simulink model "WEankle_controllerMaarten_TimingPerturb_2018"  (R2018a)
settings: Solver=FixedStepDiscrete  StartTime=0.0  StopTime=inf  FixedStep=sampleTime  RelTol=1e-3
undefined symbols (not defined in the file or in its folder): DiscIntNeverNeededParam, forceplate
libraries: simulink x17, WE2_library x8, dspsigops x6, dspfdesign x3
(part 2 of 3)

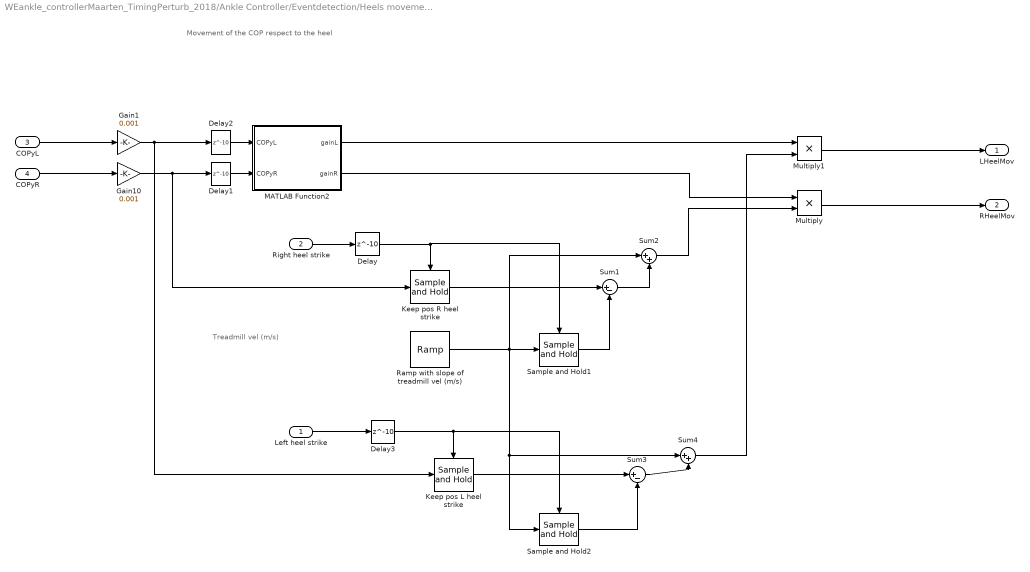
== system WEankle_controllerMaarten_TimingPerturb_2018/Ankle Controller/Eventdetection/Heels movement ==
  note: Movement of the COP respect to the heel
  note: Treadmill vel (m/s)
  Left heel strike : Inport
  Right heel strike : Inport  Port=2
  COPyL : Inport  Port=3
  COPyR : Inport  Port=4
  Delay{,1..3} (4 alike) : Delay  DelayLength=10
  Gain1 : Gain  Gain=0.001
  Gain10 : Gain  Gain=0.001
  Keep pos L heel strike : dspsigops/Sample and Hold  trig=Rising edge  initCond=0  latchinput=off
  Keep pos R heel strike : dspsigops/Sample and Hold  trig=Rising edge  initCond=0  latchinput=off
  MATLAB Function2 : MATLAB Function  TreatAsAtomicUnit=on
  Multiply : Product
  Multiply1 : Product
  Ramp with slope of treadmill vel (m/s) : simulink/Sources/Ramp  slope=-0.56  start=0  InitialOutput=0
  Sample and Hold1 : dspsigops/Sample and Hold  trig=Rising edge  initCond=0  latchinput=off
  Sample and Hold2 : dspsigops/Sample and Hold  trig=Rising edge  initCond=0  latchinput=off
  Sum1 : Sum  Inputs=|+-
  Sum2 : Sum  Inputs=|++
  Sum3 : Sum  Inputs=|+-
  Sum4 : Sum  Inputs=|++
  LHeelMov : Outport  VectorParamsAs1DForOutWhenUnconnected=off
  RHeelMov : Outport  Port=2  VectorParamsAs1DForOutWhenUnconnected=off
  wires:
  Sum2/1 -> Multiply/2
  Delay1/1 -> MATLAB Function2/2(COPyR)
  Ramp with slope of treadmill vel (m/s)/1 -> Sum4/1, Sample and Hold2/1, Sum2/1, Sample and Hold1/1
  Multiply/1 -> RHeelMov/1
  MATLAB Function2/2(gainR) -> Multiply/1
  Keep pos R heel strike/1 -> Sum1/1
  COPyR/1 -> Gain10/1
  Delay/1 -> Keep pos R heel strike/Trigger, Sample and Hold1/Trigger
  Gain10/1 -> Keep pos R heel strike/1, Delay1/1
  Sample and Hold1/1 -> Sum1/2
  Sum1/1 -> Sum2/2
  Right heel strike/1 -> Delay/1
  Delay2/1 -> MATLAB Function2/1(COPyL)
  Gain1/1 -> Delay2/1, Keep pos L heel strike/1
  COPyL/1 -> Gain1/1
  MATLAB Function2/1(gainL) -> Multiply1/1
  Left heel strike/1 -> Delay3/1
  Delay3/1 -> Sample and Hold2/Trigger, Keep pos L heel strike/Trigger
  Keep pos L heel strike/1 -> Sum3/1
  Sample and Hold2/1 -> Sum3/2
  Sum3/1 -> Sum4/2
  Sum4/1 -> Multiply1/2
  Multiply1/1 -> LHeelMov/1

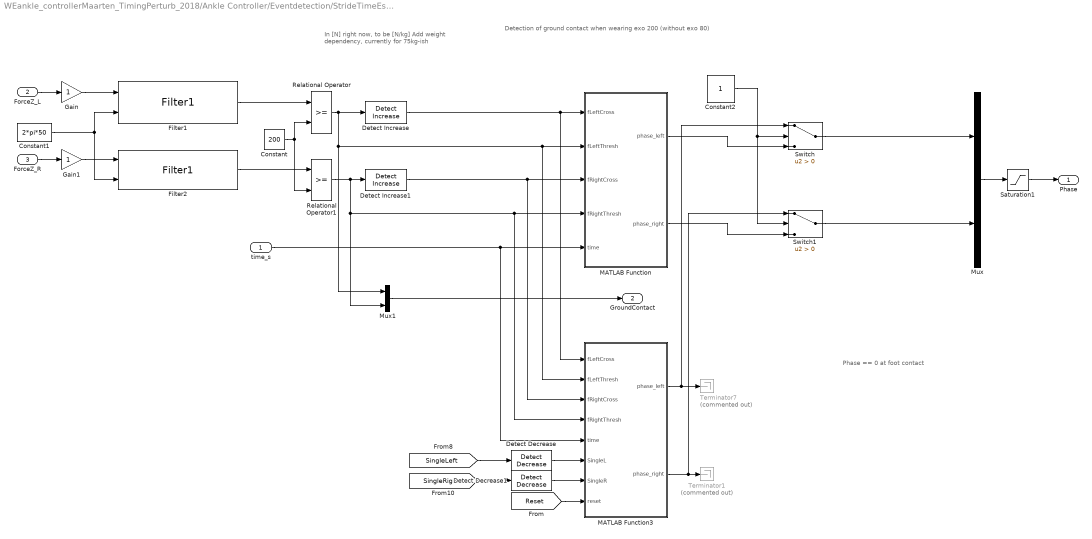
== system WEankle_controllerMaarten_TimingPerturb_2018/Ankle Controller/Eventdetection/StrideTimeEstimator ==
  note: In [N] right now, to be [N/kg]
      | Add weight dependency, currently for 75kg-ish
  note: Detection of ground contact when wearing exo 200 (without exo 80)
  note: Phase == 0 at foot contact
  time_s : Inport
  ForceZ_L : Inport  Port=2
  ForceZ_R : Inport  Port=3
  Constant : Constant  Value=200
  Constant1 : Constant  Value=2*pi*50
  Constant2 : Constant  VectorParams1D=off  SampleTime=-1
  Detect Decrease : simulink/Logic and Bit Operations/Detect Decrease  vinit=0.0  OutDataTypeStr=boolean
  Detect Decrease1 : simulink/Logic and Bit Operations/Detect Decrease  vinit=0.0  OutDataTypeStr=boolean
  Detect Increase : simulink/Logic and Bit Operations/Detect Increase  vinit=0.0  OutDataTypeStr=boolean
  Detect Increase1 : simulink/Logic and Bit Operations/Detect Increase  vinit=0.0  OutDataTypeStr=boolean
  Filter1 : WE2_library/FromActuator/ToJointAngle_rad/FilterFourthOrder/Filter1  sampleTime=sampleTime
  Filter2 : WE2_library/FromActuator/ToJointAngle_rad/FilterFourthOrder/Filter1  sampleTime=sampleTime
  Gain : Gain
  Gain1 : Gain
  MATLAB Function : MATLAB Function  TreatAsAtomicUnit=on
  MATLAB Function3 : MATLAB Function  TreatAsAtomicUnit=on
  Mux : Mux  Inputs=2
  Mux1 : Mux  Inputs=2
  Relational Operator : RelationalOperator  OutDataTypeStr=boolean  RndMeth=Simplest
  Relational Operator1 : RelationalOperator  OutDataTypeStr=boolean  RndMeth=Simplest
  Saturation1 : Saturate  UpperLimit=100  LowerLimit=0
  Switch : Switch  Criteria=u2 > Threshold
  Switch1 : Switch  Criteria=u2 > Threshold
  Terminator1 : Terminator  Commented=on
  Terminator7 : Terminator  Commented=on
  Phase : Outport  VectorParamsAs1DForOutWhenUnconnected=off
  GroundContact : Outport  Port=2  VectorParamsAs1DForOutWhenUnconnected=off
  wires:
  Gain1/1 -> Filter2/1
  Gain/1 -> Filter1/1
  Constant1/1 -> Filter1/2, Filter2/2
  Filter1/1 -> Relational Operator/1
  Filter2/1 -> Relational Operator1/1
  Mux1/1 -> GroundContact/1
  Mux/1 -> Saturation1/1
  Saturation1/1 -> Phase/1
  Switch/1 -> Mux/1
  Detect Increase1/1 -> MATLAB Function3/3(fRightCross), MATLAB Function/3(fRightCross)
  Detect Increase/1 -> MATLAB Function3/1(fLeftCross), MATLAB Function/1(fLeftCross)
  Relational Operator1/1 -> Detect Increase1/1, MATLAB Function3/4(fRightThresh), MATLAB Function/4(fRightThresh), Mux1/2
  Relational Operator/1 -> Detect Increase/1, MATLAB Function3/2(fLeftThresh), MATLAB Function/2(fLeftThresh), Mux1/1
  Constant/1 -> Relational Operator1/2, Relational Operator/2
  time_s/1 -> MATLAB Function3/5(time), MATLAB Function/5(time)
  ForceZ_R/1 -> Gain1/1
  ForceZ_L/1 -> Gain/1
  Detect Decrease/1 -> MATLAB Function3/6(SingleL)
  Detect Decrease1/1 -> MATLAB Function3/7(SingleR)
  [SingleRight] -> Detect Decrease1/1
  [SingleLeft] -> Detect Decrease/1
  MATLAB Function3/1(phase_left) -> Switch/1, Terminator7/1
  MATLAB Function3/2(phase_right) -> Switch1/1, Terminator1/1
  Switch1/1 -> Mux/2
  MATLAB Function/2(phase_right) -> Switch1/3
  MATLAB Function/1(phase_left) -> Switch/3
  Constant2/1 -> Switch1/2, Switch/2
  [Reset] -> MATLAB Function3/8(reset)

== system WEankle_controllerMaarten_TimingPerturb_2018/Ankle Controller/Eventdetection/Subsystem ==
  In1 : Inport
  Constant : Constant  Value=5
  Delay2 : Delay  DelayLength=1
  Lowpass Filter2 : dspfdesign/Lowpass Filter  FilterType=IIR  DesignForMinimumOrder=on  FilterOrder=50  PassbandFrequency=40  StopbandFrequency=50  PassbandRipple=0.1  StopbandAttenuation=40  InheritSampleRate=off  SampleRate=1000  SimulateUsing=Interpreted execution  roundingMode=Floor  coeffsDataTypeStr=fixdt(1,16)
  MATLAB Function : MATLAB Function  TreatAsAtomicUnit=on
  Rate Transition : RateTransition
  Out1 : Outport  VectorParamsAs1DForOutWhenUnconnected=off
  wires:
  MATLAB Function/1(y) -> Out1/1
  Rate Transition/1 -> Lowpass Filter2/1
  Constant/1 -> MATLAB Function/4(th)
  Lowpass Filter2/1 -> MATLAB Function/1(f)  "prev"
  Delay2/1 -> MATLAB Function/3(nf_1)
  In1/1 -> Delay2/1, MATLAB Function/2(nf), Rate Transition/1

== system WEankle_controllerMaarten_TimingPerturb_2018/Ankle Controller/Eventdetection/Subsystem1 ==
  In1 : Inport
  Constant : Constant  Value=5
  Delay2 : Delay  DelayLength=1
  Lowpass Filter2 : dspfdesign/Lowpass Filter  FilterType=IIR  DesignForMinimumOrder=on  FilterOrder=50  PassbandFrequency=40  StopbandFrequency=50  PassbandRipple=0.1  StopbandAttenuation=40  InheritSampleRate=off  SampleRate=1000  SimulateUsing=Interpreted execution  roundingMode=Floor  coeffsDataTypeStr=fixdt(1,16)
  MATLAB Function : MATLAB Function  TreatAsAtomicUnit=on
  Rate Transition : RateTransition
  Out1 : Outport  VectorParamsAs1DForOutWhenUnconnected=off
  wires:
  MATLAB Function/1(y) -> Out1/1
  Rate Transition/1 -> Lowpass Filter2/1
  Constant/1 -> MATLAB Function/4(th)
  Lowpass Filter2/1 -> MATLAB Function/1(f)  "prev"
  Delay2/1 -> MATLAB Function/3(nf_1)
  In1/1 -> Delay2/1, MATLAB Function/2(nf), Rate Transition/1

== system WEankle_controllerMaarten_TimingPerturb_2018/Ankle Controller/COMverror and perturbation/COMvError/Data lost detection ==
  note: Assuming no data lost
  Input signal : Inport
  ErrorIn : Inport  Port=2
  Delay : Delay  DelayLength=1
  Delay1 : Delay  DelayLength=1
  Gain1 : Gain  Gain=0
  Gain2 : Gain  Gain=100
  MATLAB Function1 : MATLAB Function  TreatAsAtomicUnit=on
  MATLAB Function2 : MATLAB Function  TreatAsAtomicUnit=on
  New error : Outport  VectorParamsAs1DForOutWhenUnconnected=off
  DataLost : Outport  Port=2  VectorParamsAs1DForOutWhenUnconnected=off
  avoid : Outport  Port=3  VectorParamsAs1DForOutWhenUnconnected=off
  wires:
  MATLAB Function2/2(avoid) -> avoid/1
  ErrorIn/1 -> MATLAB Function2/3(ErrorIn)
  Delay/1 -> MATLAB Function1/2(u_1)
  MATLAB Function2/1(ErrorOut) -> New error/1  "New error"
  Delay1/1 -> MATLAB Function2/2(DataLost_1)
  Input signal/1 -> MATLAB Function1/1(u), Delay/1
  MATLAB Function1/1(y) -> Gain1/1
  Gain2/1 -> DataLost/1  "DataLost"
  Gain1/1 -> Delay1/1, MATLAB Function2/1(DataLost), Gain2/1  "DataLost"

== system WEankle_controllerMaarten_TimingPerturb_2018/Ankle Controller/COMverror and perturbation/COMvError/PertDetection ==
  PertFromError : Inport
  PertFromInputSignal : Inport  Port=2
  avoid : Inport  Port=3
  Delay : Delay  DelayLength=1
  Detect Increase : simulink/Logic and Bit Operations/Detect Increase  vinit=0  OutDataTypeStr=boolean
  MATLAB Function1 : MATLAB Function  TreatAsAtomicUnit=on
  MATLAB Function2 : MATLAB Function  TreatAsAtomicUnit=on
  PertDetect : Outport  VectorParamsAs1DForOutWhenUnconnected=off
  wires:
  Detect Increase/1 -> MATLAB Function1/4(StartPertFromError)
  Delay/1 -> MATLAB Function2/2(Pert_1)
  MATLAB Function1/1(PertDetect) -> Delay/1, MATLAB Function2/1(Pert)
  PertFromInputSignal/1 -> MATLAB Function1/2(PertFromInput)
  MATLAB Function2/1(PertDetect) -> PertDetect/1
  PertFromError/1 -> MATLAB Function1/1(PertFromError), Detect Increase/1
  avoid/1 -> MATLAB Function1/3(avoid)

== system WEankle_controllerMaarten_TimingPerturb_2018/Ankle Controller/COMverror and perturbation/COMvError/Signal learner ==
  note: To convert pos to vel
  note: Excluding for the average those steps where a perturbation happened.
      | The threshold to calculate which steps where perturbed is taken as the
      | mean of maximums in previous steps. Avoiding DataLost and false Triggers
  Signaltime : Inport
  trigger : Inport  Port=2
  xPosCOM : Inport  Port=3
  Constant : Constant  Value=6
  Constant1 : Constant  Value=1.5
  Discrete Derivative1 : simulink/Discrete/Discrete Derivative  gainval=1.0  ICPrevScaledInput=0.0  OutMin=[]  OutMax=[]  OutDataType=fixdt(1, 16)  OutScaling=2^-10  DoSatur=off
  Lowpass Filter2 : dspfdesign/Lowpass Filter  FilterType=IIR  DesignForMinimumOrder=on  FilterOrder=50  PassbandFrequency=5  StopbandFrequency=50  PassbandRipple=0.1  StopbandAttenuation=40  InheritSampleRate=off  SampleRate=1000  SimulateUsing=Interpreted execution  roundingMode=Floor  coeffsDataTypeStr=fixdt(1,16)
  MATLAB Function : MATLAB Function  TreatAsAtomicUnit=on
  Rate Transition : RateTransition
  Sum : Sum  Inputs=|+-
  original : Outport  VectorParamsAs1DForOutWhenUnconnected=off
  error : Outport  Port=2  VectorParamsAs1DForOutWhenUnconnected=off
  Input filtered : Outport  Port=3  VectorParamsAs1DForOutWhenUnconnected=off
  learned : Outport  Port=4  VectorParamsAs1DForOutWhenUnconnected=off
  Perturbation detected FromInput : Outport  Port=5  VectorParamsAs1DForOutWhenUnconnected=off
  ShutDown : Outport  Port=6  VectorParamsAs1DForOutWhenUnconnected=off
  tag scope: m=global, n=global, n_strides=global, stride_duration=global
  wires:
  MATLAB Function/7(ShutDown) -> ShutDown/1
  [DataLost] -> MATLAB Function/7(DataLost)  "DataLost"
  Constant1/1 -> MATLAB Function/6(threshPert)
  MATLAB Function/6(perturbation) -> Perturbation detected FromInput/1
  trigger/1 -> MATLAB Function/3(trigger)
  Sum/1 -> error/1  "error"
  Signaltime/1 -> MATLAB Function/2(t)
  MATLAB Function/5(output_duration_) -> [stride_duration]  "stride_duration"
  Constant/1 -> MATLAB Function/5(n_rep)
  MATLAB Function/4(m_) -> [m]  "m"
  MATLAB Function/1(signal_learned) -> Sum/2, learned/1  "learned"
  MATLAB Function/2(n_strides_) -> [n_strides]  "n_strides"
  MATLAB Function/3(n_) -> [n]  "n"
  Lowpass Filter2/1 -> Sum/1, Input filtered/1, MATLAB Function/4(signal)  "prev"
  xPosCOM/1 -> Discrete Derivative1/1  "original"
  Discrete Derivative1/1 -> Rate Transition/1  "original"
  Rate Transition/1 -> original/1, Lowpass Filter2/1
  [Reset] -> MATLAB Function/1(reset)

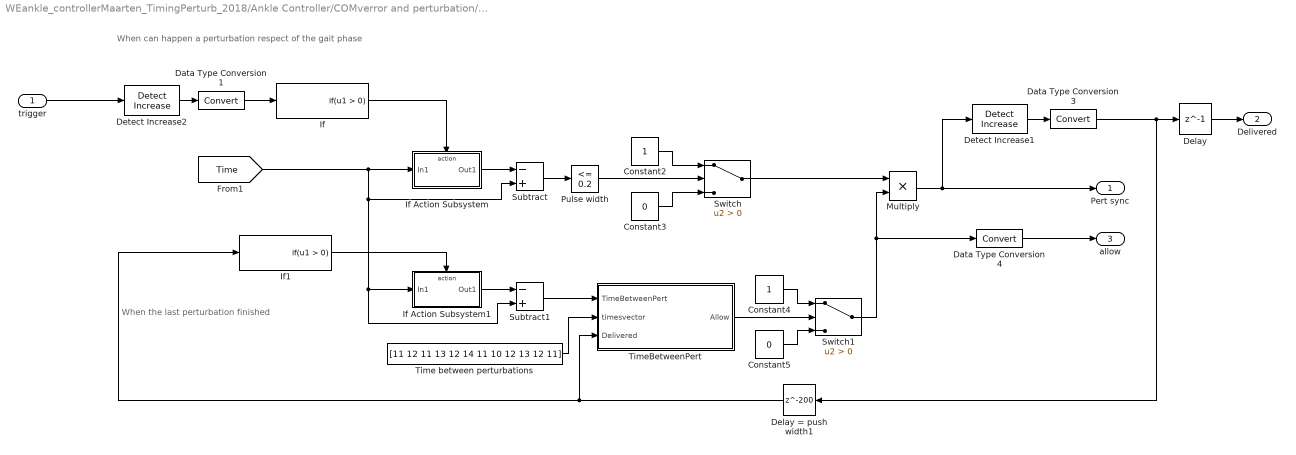
== system WEankle_controllerMaarten_TimingPerturb_2018/Ankle Controller/COMverror and perturbation/TriggerPerturbation/Perturbation sync gait phase1 ==
  note: When the last perturbation finished
  note: When can happen a perturbation respect of the gait phase
  trigger : Inport
  Constant2 : Constant
  Constant3 : Constant  Value=0
  Constant4 : Constant
  Constant5 : Constant  Value=0
  Data Type Conversion1 : DataTypeConversion
  Data Type Conversion3 : DataTypeConversion
  Data Type Conversion4 : DataTypeConversion
  Delay : Delay  DelayLength=1
  Delay = push width1 : Delay  DelayLength=200  InitialCondition=0
  Detect Increase1 : simulink/Logic and Bit Operations/Detect Increase  vinit=0  OutDataTypeStr=boolean
  Detect Increase2 : simulink/Logic and Bit Operations/Detect Increase  vinit=0  OutDataTypeStr=boolean
  If : If  ShowElse=off
  If Action Subsystem : Subsystem  TreatAsAtomicUnit=on
  If Action Subsystem1 : Subsystem  TreatAsAtomicUnit=on
  If1 : If  ShowElse=off
  Multiply : Product
  Pulse width : simulink/Logic and Bit Operations/Compare To Constant  relop=<=  const=0.2  OutDataTypeStr=boolean
  Subtract : Sum  Inputs=-+
  Subtract1 : Sum  Inputs=-+
  Switch : Switch  Criteria=u2 > Threshold
  Switch1 : Switch  Criteria=u2 > Threshold
  Time between perturbations : Constant  Value=[11 12 11 13 12 14 11 10 12 13 12 11]
  TimeBetweenPert : MATLAB Function  TreatAsAtomicUnit=on
  Pert sync : Outport  VectorParamsAs1DForOutWhenUnconnected=off
  Delivered : Outport  Port=2  VectorParamsAs1DForOutWhenUnconnected=off
  allow : Outport  Port=3  VectorParamsAs1DForOutWhenUnconnected=off
  wires:
  Time between perturbations/1 -> TimeBetweenPert/2(timesvector)
  Subtract1/1 -> TimeBetweenPert/1(TimeBetweenPert)
  TimeBetweenPert/1(Allow) -> Switch1/2
  Data Type Conversion4/1 -> allow/1
  Delay/1 -> Delivered/1
  Data Type Conversion3/1 -> Delay/1, Delay = push width1/1
  Delay = push width1/1 -> If1/1, TimeBetweenPert/3(Delivered)
  If1/1 -> If Action Subsystem1/Action
  Constant3/1 -> Switch/3
  If/1 -> If Action Subsystem/Action
  Constant2/1 -> Switch/1
  [Time] -> Subtract1/2, If Action Subsystem1/1(In1), Subtract/2, If Action Subsystem/1(In1)
  Constant5/1 -> Switch1/3
  Pulse width/1 -> Switch/2
  Multiply/1 -> Detect Increase1/1, Pert sync/1
  If Action Subsystem/1(Out1) -> Subtract/1
  If Action Subsystem1/1(Out1) -> Subtract1/1
  trigger/1 -> Detect Increase2/1
  Subtract/1 -> Pulse width/1
  Switch/1 -> Multiply/1
  Switch1/1 -> Multiply/2, Data Type Conversion4/1
  Detect Increase2/1 -> Data Type Conversion1/1
  Data Type Conversion1/1 -> If/1
  Constant4/1 -> Switch1/1
  Detect Increase1/1 -> Data Type Conversion3/1

== system WEankle_controllerMaarten_TimingPerturb_2018/Ankle Controller/Eventdetection/COP detection (treadmill)/Get_COPL ==
  note: COPx
  note: COPy
  grf : Inport
  Enable : EnablePort  StatesWhenEnabling=reset
  Demux1 : Demux  Outputs=3
  Divide : Product  Inputs=*/
  Divide1 : Product  Inputs=*/
  Gain : Gain  Gain=-1
  LEFT Mx My Fz : Selector  InputPortWidth=6  IndexOptions=Index vector (dialog)  Indices=[4 5 3]  OutputSizes=1
  Mux : Mux  Inputs=2
  COPL : Outport  OutputWhenDisabled=reset  InitialOutput=0  VectorParamsAs1DForOutWhenUnconnected=off
  wires:
  grf/1 -> LEFT Mx My Fz/1
  LEFT Mx My Fz/1 -> Demux1/1
  Demux1/2 -> Gain/1  "My"
  Gain/1 -> Divide/1
  Demux1/3 -> Divide1/2, Divide/2  "Fz"
  Demux1/1 -> Divide1/1  "Mx"
  Divide/1 -> Mux/1
  Divide1/1 -> Mux/2
  Mux/1 -> COPL/1

== system WEankle_controllerMaarten_TimingPerturb_2018/Ankle Controller/Eventdetection/COP detection (treadmill)/Get_COPR ==
  note: COPx
  note: COPy
  grf : Inport
  Enable : EnablePort  StatesWhenEnabling=reset
  Demux1 : Demux  Outputs=3
  Divide : Product  Inputs=*/
  Divide1 : Product  Inputs=*/
  Gain : Gain  Gain=-1
  Mux : Mux  Inputs=2
  RIGHT Mx My Fz : Selector  InputPortWidth=6  IndexOptions=Index vector (dialog)  Indices=[4 5 3]  OutputSizes=1
  COPR : Outport  OutputWhenDisabled=reset  InitialOutput=0  VectorParamsAs1DForOutWhenUnconnected=off
  wires:
  grf/1 -> RIGHT Mx My Fz/1
  RIGHT Mx My Fz/1 -> Demux1/1
  Demux1/2 -> Gain/1  "My"
  Gain/1 -> Divide/1
  Demux1/3 -> Divide1/2, Divide/2  "Fz"
  Demux1/1 -> Divide1/1  "Mx"
  Divide/1 -> Mux/1
  Divide1/1 -> Mux/2
  Mux/1 -> COPR/1

== system WEankle_controllerMaarten_TimingPerturb_2018/Ankle Controller/COMverror and perturbation/TriggerPerturbation/Perturbation sync gait phase1/If Action Subsystem ==
  In1 : Inport
  Action Port : ActionPort
  Out1 : Outport  VectorParamsAs1DForOutWhenUnconnected=off
  wires:
  In1/1 -> Out1/1

== system WEankle_controllerMaarten_TimingPerturb_2018/Ankle Controller/COMverror and perturbation/TriggerPerturbation/Perturbation sync gait phase1/If Action Subsystem1 ==
  In1 : Inport
  Action Port : ActionPort
  Out1 : Outport  VectorParamsAs1DForOutWhenUnconnected=off
  wires:
  In1/1 -> Out1/1

== matlab function WEankle_controllerMaarten_TimingPerturb_2018/Ankle Controller/Eventdetection/StrideTimeEstimator/MATLAB Function ==
  data: fLeftCross input; fLeftThresh input; phase_left output; fRightCross input; fRightThresh input; time input; phase_right output
function [phase_left, phase_right] = fcn(fLeftCross, fLeftThresh, fRightCross, fRightThresh, time)

persistent time_heel2heel_right
persistent time_heellast_right
persistent tdm_right
persistent time_heel2heel_left
persistent time_heellast_left
persistent tdm_left

if(isempty(time_heel2heel_left))
   time_heel2heel_right = zeros(4,1);
   time_heellast_right = -1e5;
   tdm_right = 0.1;
   
   time_heel2heel_left = zeros(4,1);
   time_heellast_left = -1e5;
   tdm_left = 0.1;
end
%% left
phase_left = (time - time_heellast_left)/(tdm_left+eps)*100;
if(fLeftCross~=0||(phase_left>100&&fLeftThresh==1))
    td_new  = time - time_heellast_left;
    if((td_new>0.8*tdm_left)||any(time_heel2heel_left>10))
        time_heellast_left = time;
        time_heel2heel_left(2:end) = time_heel2heel_left(1:end-1);
        time_heel2heel_left(1) = td_new;
        tdm_left = mean(time_heel2heel_left);
    end
end


%% right
phase_right = (time - time_heellast_right)/(tdm_right+eps)*100;
if(fRightCross~=0||(phase_right>100&&fRightThresh==1))
    td_new  = time - time_heellast_right;
    if((td_new>0.8*tdm_right)||any(time_heel2heel_right>10))
        time_heellast_right = time;
        time_heel2heel_right(2:end) = time_heel2heel_right(1:end-1);
        time_heel2heel_right(1) = td_new;
        tdm_right = mean(time_heel2heel_right);
    end
end

== matlab function WEankle_controllerMaarten_TimingPerturb_2018/Ankle Controller/Eventdetection/COP detection (treadmill)/MATLAB Function1 ==
  data: x input; y output; OmegaFilter input; sampleTime input
function y = Filter2ndOrder(x, OmegaFilter, sampleTime)
%#codegen

persistent yd_prev y_prev;
if isempty(yd_prev)
    yd_prev = zeros(6,1); 
    y_prev = zeros(6,1);  %Derivative of the above signal
end

% Do 2nd order filtering with given omega and zeta=0.7; input of filter
% is vel_inc_sampleTime_unfilt; output is y (we assign to vel_inc_s
% later). 
if OmegaFilter==0 || isinf(OmegaFilter)
    y = x;
    y_prev = y;
    yd_prev = zeros(6,1); 
else
    zeta = 0.7;
    ydd = OmegaFilter^2 * (x - y_prev) - 2*zeta*OmegaFilter* yd_prev;
    yd = yd_prev + ydd * sampleTime;
    y = y_prev + yd * sampleTime;

    y_prev = y; yd_prev = yd;
end

== matlab function WEankle_controllerMaarten_TimingPerturb_2018/Ankle Controller/MATLAB Function5 ==
  data: e0 input; G input; SolGains output; COMd input
function SolGains  = CombineSoleusGains(e0,G,COMd)
% input arguments:

SolGains = [e0; G; COMd];

== matlab function WEankle_controllerMaarten_TimingPerturb_2018/ForcePlate/Calibration/MATLAB Function ==
  data: left input; left_calib output; right input; start input; right_calib output; caltime_s input
function [left_calib, right_calib] = calibrateOffset(left, right, start, caltime_s)
persistent calibrated
persistent offcum_left
persistent offcum_right
persistent counter
persistent nosamp

if(isempty(calibrated))
   calibrated = false;
   offcum_left = left*0;
   offcum_right = right*0;
   counter = 0;
   nosamp = max(1, floor(caltime_s*1000));
end

if(start == 1)
    counter = 0;
    calibrated = false;
    offcum_left = left*0;
    offcum_right = right*0;
    nosamp = max(1, floor(caltime_s*1000));
end

if(calibrated)
    left_calib = left - offcum_left;
    right_calib = right - offcum_right;
else
    if(~calibrated)
        counter = counter + 1;
        offcum_left = offcum_left + left/(nosamp);
        offcum_right = offcum_right + right/(nosamp);
        if(counter >= nosamp)
            calibrated = true;
        end
    end
    left_calib = left;
    right_calib = right;
end

== matlab function WEankle_controllerMaarten_TimingPerturb_2018/Ankle Controller/Eventdetection/COP detection (treadmill)/MATLAB Function2 ==
  data: x input; y output; OmegaFilter input; sampleTime input
function y = Filter2ndOrder(x, OmegaFilter, sampleTime)
%#codegen

persistent yd_prev y_prev;
if isempty(yd_prev)
    yd_prev = zeros(6,1); 
    y_prev = zeros(6,1);  %Derivative of the above signal
end

% Do 2nd order filtering with given omega and zeta=0.7; input of filter
% is vel_inc_sampleTime_unfilt; output is y (we assign to vel_inc_s
% later). 
if OmegaFilter==0 || isinf(OmegaFilter)
    y = x;
    y_prev = y;
    yd_prev = zeros(6,1); 
else
    zeta = 0.7;
    ydd = OmegaFilter^2 * (x - y_prev) - 2*zeta*OmegaFilter* yd_prev;
    yd = yd_prev + ydd * sampleTime;
    y = y_prev + yd * sampleTime;

    y_prev = y; yd_prev = yd;
end

== matlab function WEankle_controllerMaarten_TimingPerturb_2018/Ankle Controller/COMverror and perturbation/TriggerPerturbation/Perturbation sync gait phase1/TimeBetweenPert ==
  data: TimeBetweenPert input; timesvector input; Allow output; Delivered input
function Allow = fcn(TimeBetweenPert,timesvector,Delivered)
% To randomize the time between perturbations (min 6s)
persistent i 
persistent TimeSelector 
persistent flagfirst %flag to indicate first time
if isempty(i)
    i = 1;
    flagfirst = 1;
end
if Delivered == 1 && ~flagfirst %Perturbation delivered. Go to next element of timesVector avoiding a false entrance the first time
    i = i+1;
end
%% Assign new time
len = length(timesvector);
if i > len %reset the index when all perturbations from the vector are done
    i = 1;
end
TimeSelector = timesvector(i);

if TimeSelector < 6
    TimeSelector = 6;
end
%% Allow new perturbation or not
if TimeBetweenPert >= TimeSelector
    Allow = 1;
else
    Allow = 0;
end
%%
flagfirst = 0;

== matlab function WEankle_controllerMaarten_TimingPerturb_2018/Ankle Controller/Eventdetection/Subsystem/MATLAB Function ==
  data: f input; y output; nf input; nf_1 input; th input
function y = fcn(f,nf,nf_1,th)

maxCounter = 200; %time to wait in zero
persistent counter
persistent out
if isempty(counter)
    counter = maxCounter+1;
    out = f;
end

if (nf == 0) && (nf_1 < -50)
    out = 0;
    counter = 0;
else
    counter = counter+1;
    if counter > maxCounter
        if (f > -th) && (f < th) && (nf == 0)
            out = 0;
        else
            out = f;
        end
    end
end

y = out;

== matlab function WEankle_controllerMaarten_TimingPerturb_2018/Ankle Controller/Eventdetection/StrideTimeEstimator/MATLAB Function3 ==
  data: fLeftCross input; fLeftThresh input; phase_left output; fRightCross input; fRightThresh input; time input; phase_right output; SingleL input; SingleR input; reset input
function [phase_left, phase_right] = fcn(fLeftCross, fLeftThresh, fRightCross, fRightThresh, time, SingleL, SingleR, reset)

persistent time_heel2heel_right
persistent time_heellast_right
persistent tdm_right
persistent time_heel2heel_left
persistent time_heellast_left
persistent tdm_left
persistent  phase_left2
persistent  phase_right2

if(isempty(time_heel2heel_left) || reset==1)
   time_heel2heel_right = zeros(4,1);
   time_heellast_right = -1e5;
   tdm_right = 0.1;
   
   time_heel2heel_left = zeros(4,1);
   time_heellast_left = -1e5;
   tdm_left = 0.1;
   
    phase_left2 = 0; %Used to reset the left phase when prepositioning of left leg is detected (SingleL 1 to 0)
    phase_right2 = 0; %Used to reset the right phase when prepositioning of right leg is detected (SingleR 1 to 0)
end
%% left
phase_left = (time - time_heellast_left)/(tdm_left+eps)*100 - phase_left2;
% if(fLeftCross~=0||(phase_left>100&&fLeftThresh==1))

if(SingleR)
    phase_left2 = phase_left;
end
if((fLeftCross~=0||(phase_left>100&&fLeftThresh==1)))
    td_new  = time - time_heellast_left;
    phase_left2 = 0;
    if((td_new>0.8*tdm_left)||any(time_heel2heel_left>10))
        time_heellast_left = time;
        time_heel2heel_left(2:end) = time_heel2heel_left(1:end-1);
        time_heel2heel_left(1) = td_new;
        tdm_left = mean(time_heel2heel_left);
    end
end


%% right
phase_right = (time - time_heellast_right)/(tdm_right+eps)*100 - phase_right2;
% if(fRightCross~=0||(phase_right>100&&fRightThresh==1))
if(SingleL)
    phase_right2 = phase_right;
end
if(fRightCross~=0||(phase_right>100&&fRightThresh==1))
    td_new  = time - time_heellast_right;
    phase_right2 = 0;
    if((td_new>0.8*tdm_right)||any(time_heel2heel_right>10))
        time_heellast_right = time;
        time_heel2heel_right(2:end) = time_heel2heel_right(1:end-1);
        time_heel2heel_right(1) = td_new;
        tdm_right = mean(time_heel2heel_right);
    end
end

== matlab function WEankle_controllerMaarten_TimingPerturb_2018/Merge 32 bit to double/MATLAB Function ==
  data: time_0 input; unix_time output double size=1; time_1 input int32 size=1
function unix_time  = fcn(time_0, time_1)

% Convert both integers to double, scale up the most significant part and
% add them together.
% The epoch is also moved from 1601 to 1970, this is done in the integer
% part.

double_0 = double(time_0);
double_1 = double(time_1 - int32(27111902));
unix_time = (double_1 * 2^32 + double_0 - 3577643008.0) * 1.0e-7;

% A 64 bit integer does not exist in Simulink 2018b. Casting is also not
% possible, otherwise the following would work:
% time_64bit = typecast([time_0, time_1], 'int64');
% unix_time = double(time_64bit);

end

== matlab function WEankle_controllerMaarten_TimingPerturb_2018/Ankle Controller/COMverror and perturbation/TriggerPerturbation/MakeVect ==
  data: u input; y output
function y = fcn(u)

y = [u, u, u, u, u];

== matlab function WEankle_controllerMaarten_TimingPerturb_2018/Ankle Controller/COMDLimits ==
  data: comd input; comd_out output
function comd_out = COMd_bounds(comd)


tresh = 200; % 200mm/s

if abs(comd)<tresh    
    comd = 0;
end


comd_out = comd;

== matlab function WEankle_controllerMaarten_TimingPerturb_2018/Ankle Controller/Eventdetection/Heels movement/MATLAB Function2 ==
  data: gainL output; COPyL input; gainR output; COPyR input
function [gainL,gainR] = Stance(COPyL,COPyR)
%#codegen
if COPyR == 0
    gainR = 0;
else
    gainR = 1;
end

if COPyL == 0
    gainL = 0;
else
    gainL = 1;
end

end

== matlab function WEankle_controllerMaarten_TimingPerturb_2018/Ankle Controller/COMverror and perturbation/TriggerPerturbation/PushOrPull ==
  data: Perturb input; vectorPushPull input; NewPert output; Delivered input
function NewPert = fcn(Perturb,vectorPushPull,Delivered)
% To randomize pushes and pulls
persistent i 
persistent Selector 
persistent flagfirst %flag to indicate first time
if isempty(i)
    i = 1;
    flagfirst = 1;
end
if Delivered == 1 && ~flagfirst %Perturbation delivered. Go to next element of timesVector avoiding a false entrance the first time
    i = i+1;
end
%%
len = length(vectorPushPull);
if i > len %reset the index when all perturbations from the vector are done
    i = 1;
end
Selector = vectorPushPull(i);

if Selector < -1
    Selector = -1;
elseif Selector > 1
    Selector = 1;
end
%% 
NewPert = Selector*Perturb;
%%
flagfirst = 0;

== matlab function WEankle_controllerMaarten_TimingPerturb_2018/Ankle Controller/COMverror and perturbation/COMvError/MATLAB Function1 ==
  data: ShutDown input; PertDetect input; TriggerPush output
function TriggerPush = fcn(ShutDown,PertDetect)
if ShutDown == 0
    TriggerPush = PertDetect;
else
    TriggerPush = 0;
end

== matlab function WEankle_controllerMaarten_TimingPerturb_2018/Ankle Controller/COMverror and perturbation/COMvError/Signal learner/MATLAB Function ==
  data: reset input; t input; trigger input; signal input; signal_learned output; n_strides_ output; n_ output; m_ output; output_duration_ output; n_rep input; perturbation output; threshPert input; DataLost input; ShutDown output
function [signal_learned,n_strides_,n_,m_,output_duration_,perturbation,ShutDown] = signal_learner(reset,t,trigger,signal,n_rep,threshPert,DataLost)
%     n_rep = how many signals period will be averaged
n_storage = 2000; %stored signal will be 2000 elements long. playback will be interpolated
n_buffer_size = 4000; %can maximally read 4000;
perturbation = 0;
ShutDown = 0; %No trigger the controller if DataLost or if we are in the first n_rep strides
persistent n %elements of vector
persistent n_strides % total number of strides
persistent m %Pointer for recording each stride in buffer (1:n_rep)
persistent t0 % moment in time of last stride
persistent last_buffer
persistent output_signal_buffer
persistent output_signal
persistent output_duration
persistent output_duration_buffer
persistent maximums
persistent MaxAver
persistent LastTrigger



if isempty(n)
    n = 1;
    m = 1;
    t0 = 0;
    last_buffer = zeros(1,n_buffer_size);
    output_signal_buffer = zeros(n_rep,n_storage);
    output_signal = zeros(1,n_storage);
    output_duration_buffer = zeros(n_rep,1);
    n_strides = 0;
    output_duration = 1;
    % Added Cristina
    maximums = 200*ones(n_rep,1); %to store the maximums of previous steps
    MaxAver = 200; % This number multiplied by 1.5 is the one above which a perturbation is supposed to happen,
    %     and thereby, that step will be excluded to calculate the mean
    LastTrigger = 0;
end

dtStride = t-LastTrigger;
if trigger
    LastTrigger = t;
end

if dtStride <0.1 || dtStride > 4
    reset = 1;
end



if ~DataLost && ~reset
    t_rel = t-t0;
    if (trigger && t_rel > 0.1) %if trigger happens, note down the absolute time when that was
        n_strides = n_strides+1; %counting number of strides
        last_stride_duration = t-t0;
        
        t0 = t; %Reset the moment when the last stride happened
        %% Added Cristina
        % See if there was a perturbation in the last step
        Perturbation = 0; % Init perturbation in the last step
%         leng = length(last_buffer(1:min([n,n_buffer_size])));
%         for i = 1:leng
%             element = last_buffer(i);
%             if element > 1.5*MaxAver % A perturbation was detected in the last step
%                 Perturbation = 1;
%             end
%         end
        
        %% Changed Cristina
        enter = 1;
%         if n_strides >= 3
%             if (last_stride_duration > 0.5*output_duration)% to avoid false triggers
%                 enter = 1;
%             else
%                 enter = 0;
%             end
%         else
%             enter = 1;
%         end
        if (last_stride_duration > 0) && enter % otherwise failure at start or false trigger  
            % If there was no perturbation, take that step into account.
            % Otherwise, exclude it
            if ~Perturbation %in the last step
                %interpolate regardless of last duration to n_storage elements
%                 if n == 1
%                     n = n+1;
%                 end
                output_signal_buffer(m,:) = ...
                    interp1(...
                    linspace(0,last_stride_duration,n),... %vector of n elements
                    last_buffer(1:min([n,n_buffer_size])),... %only read up to incl. n elements, if bigger than n_buffer size, then we need to limit.
                    linspace(0,last_stride_duration,n_storage)); %remap that to a new 'x' with n_storage elements
                output_signal = mean(output_signal_buffer); %averages over n_rep stored signals
                
                output_duration_buffer(m) = last_stride_duration;
                output_duration = mean(output_duration_buffer); %duration is average of last n_rep times
                
                maximums(m) = max(last_buffer(1:min([n,n_buffer_size]))); %store the new maximum of current step
                MaxAver = mean(maximums); %calculate the average of maximums found in the last n_rep
                
                m = m+1;
                if m > n_rep
                    m = 1;
                end
            end
            if (n_strides <= n_rep)
                output_duration = last_stride_duration;
            end
            %last_buffer = zeros() %is not required due to 1:n
            n = 1;
        end
    end
end
if ~DataLost && ~reset
    %% process input
    t_rel = t-t0;
    last_buffer(min([n n_buffer_size])) = signal;
    
    %% generate output
    fractional_index = t_rel/output_duration * (n_storage-1);
    rounded_index = min([1+floor(fractional_index),n_storage]); %cannot overflow
    fraction = 1+fractional_index - rounded_index;
    
    %linearly interpolate
    if (rounded_index >= n_storage - 1)
        signal_learned = output_signal(n_storage-1);
    else
        signal_learned = output_signal(rounded_index)*(1-fraction) + output_signal(rounded_index+1)*fraction;
    end
    
    %debug output
    n_strides_ = n_strides;
    n_ = n;
    m_ = m;
    output_duration_ = output_duration;
    if signal > threshPert*MaxAver
        perturbation = 1;
    end
else
    %debug output
    n_strides_ = n_strides;
    n_ = n;
    m_ = m;
    output_duration_ = output_duration;
    perturbation = 0;
    signal_learned = 0;
end

%do not output anything learned in first n_rep strides.
if (n_strides <= n_rep) || DataLost || reset
    signal_learned = 0;
    output_duration_ = 0;%last_stride_duration;
    ShutDown = 1;
end
if ~DataLost && ~reset
    %shift signal storage pointer, avoid overflow
    n = n+1;
else
    n = 1;
end
end

== matlab function WEankle_controllerMaarten_TimingPerturb_2018/Ankle Controller/COMverror and perturbation/COMvError/Data lost detection/MATLAB Function1 ==
  data: u input; y output; u_1 input
function y = fcn(u,u_1)
% input signal u = xVelCOM
% output y = data lost detection (1 or 0)
y = 0;
if u == u_1 % The new data is equal to the previous one --> See how Qualisys will send it since NaN is not supported
    y = 1; % Data lost
else
    y = 0; % Data good
end

== matlab function WEankle_controllerMaarten_TimingPerturb_2018/Ankle Controller/COMverror and perturbation/COMvError/Data lost detection/MATLAB Function2 ==
  data: DataLost input; DataLost_1 input; ErrorOut output; ErrorIn input; avoid output
function [ErrorOut,avoid] = fcn(DataLost,DataLost_1,ErrorIn)
% ErrorOut is the new error corrected when data lost

maxCounter = 1500; %time to wait after a DataLost detection to let the controller works again (1.5s)
persistent counter
if isempty(counter)
    counter = maxCounter+1;
end

ErrorOut = ErrorIn;
avoid = 0;

if DataLost == 1 % Data lost
    ErrorOut = 0; 
    avoid = 1;
elseif DataLost == 0 && DataLost_1 == 1 % Data just recovered after a loss
    counter = 1;
    ErrorOut = 0; 
    avoid = 1;
elseif DataLost == 0 && DataLost_1 ~= 1 % Good data
    if counter <= maxCounter % Wait 1.5s after data has been recovered to generate the newError
        ErrorOut = 0;
        avoid = 1;
        counter = counter + 1;
    else
        ErrorOut = ErrorIn;
        avoid = 0;
    end
end

== matlab function WEankle_controllerMaarten_TimingPerturb_2018/Ankle Controller/COMverror and perturbation/COMvError/PerturbationDetectionFromError ==
  data: t input; trigger input; signal input; n_rep input; push output; maxAver output; rangeAver output; threshPert input; DataLost input
function [push,maxAver,rangeAver] = PerturbationDetectionFromError(t,trigger,signal,n_rep,threshPert,DataLost)
    n_buffer_size = 4000; %can maximally read 4000;
    push = 0; 
    
    persistent n %elements of vector
    persistent n_strides % total number of strides
    persistent m %Pointer for recording each stride in buffer (1:n_rep)
    persistent t0 % moment in time of last stride
    persistent last_buffer
    persistent maximums
    persistent MaxAver
    persistent minimums
    persistent MinAver
    persistent RangeAver

    if isempty(n)
       n = 1;
       m = 1;
       t0 = 0;
       last_buffer = zeros(1,n_buffer_size);
       n_strides = 0;

       maximums = 50*ones(n_rep,1); %to store the maximums of previous steps
       MaxAver = 50; % This number multiply by 1.5 is the one above which a push perturbation is supposed to happen,
%     and thereby, that step will be excluded to calculate the mean of
%     maximums
       minimums =  -120*ones(n_rep,1);
       MinAver = -120;
       RangeAver = 170;
    end
if ~DataLost
    t_rel = t-t0;
    if (trigger && t_rel > 0.1) %if trigger happens, note down the absolute time when that was
        n_strides = n_strides+1; %counting number of strides
        last_stride_duration = t-t0;

        t0 = t; %Reset the moment when the last stride happened
        %% Added Cristina
        % See if there was a perturbation in the last step
        Push = 0; % Init perturbation in the last step
        leng = length(last_buffer(1:min([n,n_buffer_size])));
        for i = 1:leng
            element = last_buffer(i);
            if element > 1.5*MaxAver % A perturbation was detected in the last step
                Push = 1;
            end
        end
        
        %% Changed Cristina
        if (last_stride_duration > 0) %otherwise failure at start
            % If there was no perturbation, take that step into account.
            % Otherwise, exclude it
            if ~Push %in the last step                
                maximums(m) = max(last_buffer(1:min([n,n_buffer_size]))); %store the new maximum of current step
                MaxAver = mean(maximums); %calculate the average of maximums found in the last n_rep
                
                minimums(m) = min(last_buffer(1:min([n,n_buffer_size]))); %store the new minimum of current step
                MinAver = mean(minimums); %calculate the average of minimums found in the last n_rep
                RangeAver = MaxAver - MinAver;
                
                m = m+1;
                if m > n_rep 
                    m = 1;
                end
            end

            n = 1;
        end
    end
end
if ~DataLost
    %% process new data
    last_buffer(min([n n_buffer_size])) = signal;
    
    %% generate output
    if signal > threshPert*RangeAver 
        push = 1;
    end
    maxAver = MaxAver;
    rangeAver = RangeAver;
    
else
    maxAver = MaxAver;
    rangeAver = RangeAver;
    push = 0;
end
%do not output anything learned in first n_rep strides.
if (n_strides <= n_rep) || DataLost
    push = 0;
end

if ~DataLost
    %shift signal storage pointer, avoid overflow
    n = n+1;
else
    n = 1;
end
end

== matlab function WEankle_controllerMaarten_TimingPerturb_2018/Ankle Controller/COMverror and perturbation/COMvError/PertDetection/MATLAB Function1 ==
  data: PertFromError input; PertDetect output; PertFromInput input; avoid input; StartPertFromError input
function PertDetect = NotTriggerIfDataLost(PertFromError,PertFromInput,avoid,StartPertFromError)
% PertFromError is already including the data lost because the error will
% be zero if that happens. But it could be that PertFromInput says there is
% a perturbation, and that is why this is needed

%avoid because data lost

persistent CounterPertError
if isempty(CounterPertError)
    CounterPertError = 0;
end
if StartPertFromError
    CounterPertError = CounterPertError +1;
end
%Discard the first two perturbations detected from error
if (PertFromError || PertFromInput) && ~avoid && (CounterPertError > 2)  %Detect a new perturbation
    PertDetect = 1;
else
    PertDetect = 0;
end

== matlab function WEankle_controllerMaarten_TimingPerturb_2018/Ankle Controller/COMverror and perturbation/COMvError/PertDetection/MATLAB Function2 ==
  data: Pert input; PertDetect output; Pert_1 input
function PertDetect = WaitForNewDetect(Pert,Pert_1)
PertDetect = 0;
% Wait 2s to trigger a new perturbation if a previous one was detected

maxCounter = 2000; %time to wait after a Perturbation detection to detect a new one
persistent counter
if isempty(counter)
    counter = maxCounter+1;
end

if Pert_1 == 0 && Pert == 1 %New possible perturbation
    if counter > maxCounter
        PertDetect = Pert;
    else
        PertDetect = 0;
    end
elseif Pert_1 == 1 && Pert == 1 %middle of a perturbation
    if counter > maxCounter
        PertDetect = Pert;
    else
        PertDetect = 0;
    end
elseif Pert_1 == 1 && Pert == 0 % end of a perturbation
    counter = 1;
    PertDetect = Pert;
end

counter = counter + 1;

== matlab function WEankle_controllerMaarten_TimingPerturb_2018/Ankle Controller/Eventdetection/Subsystem1/MATLAB Function ==
  data: f input; y output; nf input; nf_1 input; th input
function y = fcn(f,nf,nf_1,th)

maxCounter = 200; %time to wait in zero
persistent counter
persistent out
if isempty(counter)
    counter = maxCounter+1;
    out = f;
end

if (nf == 0) && (nf_1 < -50)
    out = 0;
    counter = 0;
else
    counter = counter+1;
    if counter > maxCounter
        if (f > -th) && (f < th) && (nf == 0)
            out = 0;
        else
            out = f;
        end
    end
end

y = out;

== matlab function WEankle_controllerMaarten_TimingPerturb_2018/Ankle Controller/Eventdetection/MATLAB Function2 ==
  data: COPyL input; leftFront output; COPyR input; rightFront output; singleLeft output; singleRight output; COPyL_1 input; COPyR_1 input
% function [LeftFront,RightFront,SingleLeft,SingleRight] = DetectionFrontFoot(COPyL,COPyR,COPyL_1,COPyR_1)
function [leftFront,rightFront,singleLeft,singleRight] = DetectionFrontFoot(COPyL,COPyR,COPyL_1,COPyR_1)
%#codegen
% LeftFront = 0; 
% RightFront = 0;
% SingleRight = 0;
% SingleLeft = 0;

persistent LeftFront
persistent RightFront
persistent SingleRight
persistent SingleLeft

maxCounter = 3; %time to wait to avoid false detection
maxCounterStance = 4;
persistent counter
persistent counterStance
if isempty(counter)
    counter = maxCounter+1;
    counterStance = maxCounterStance+1;
    LeftFront = 0;
    RightFront = 0;
    SingleRight = 0;
    SingleLeft = 0;
end

%%
if (COPyL~=0) && (COPyR~=0) && ((COPyL_1 == 0) || (COPyR_1 == 0)) %Possible init of double stance
    counterStance = 0;
elseif (COPyL~=0) && (COPyR~=0) && (COPyL_1 ~= 0) && (COPyR_1 ~= 0) % Possible double stance
    counterStance = counterStance + 1;
    if counterStance > maxCounterStance
        if COPyL > COPyR %Left in front
            LeftFront = 1;
            RightFront = 0;
            SingleRight = 0;
            SingleLeft = 0;
        elseif COPyL < COPyR %Rigth in front
            LeftFront = 0;
            RightFront = 1;
            SingleRight = 0;
            SingleLeft = 0;
        end
    end
    
% if (COPyL~=0) && (COPyR~=0) %Double stance
%     if COPyL > COPyR %Left in front
%         LeftFront = 1;
%         RightFront = 0;
%         SingleRight = 0;
%         SingleLeft = 0;
%     elseif COPyL < COPyR %Rigth in front
%         LeftFront = 0;
%         RightFront = 1;
%         SingleRight = 0;
%         SingleLeft = 0;
%     end
elseif (COPyL == 0) && (COPyR == 0) %No one on the treadmill
    LeftFront = 0;
    RightFront = 0;
    SingleRight = 0;
    SingleLeft = 0;
elseif (COPyL == 0) && (COPyL_1 ~= 0) && (COPyR ~= 0) %Init of a possible Left swing, Rigth stance
    counter = 0;
    LeftFront = 0;
    RightFront = 1;
elseif (COPyL == 0) && (COPyL_1 == 0) && (COPyR ~= 0) % Possible Left swing, Rigth stance
    counter = counter+1;
    LeftFront = 0;
    RightFront = 1;
    if counter > maxCounter
        SingleRight = 1;
        SingleLeft = 0;
    end
elseif (COPyR == 0) && (COPyR_1 ~= 0) && (COPyL ~= 0) %Init of a possible Right swing, Left stance
    counter = 0;
    LeftFront = 1;
    RightFront = 0;
elseif (COPyR == 0) && (COPyR_1 == 0) && (COPyL ~= 0) %Possible Right swing, Left stance
    counter = counter+1;
    LeftFront = 1;
    RightFront = 0;
    if counter > maxCounter
        SingleRight = 0;
        SingleLeft = 1;
    end
end

leftFront = LeftFront;
rightFront =RightFront; 
singleRight = SingleRight;
singleLeft = SingleLeft;
end

== matlab function WEankle_controllerMaarten_TimingPerturb_2018/Ankle Controller/MATLAB Function6 ==
  data: e0 input; G input; loff input; GSol input; TibGains output; COMd input
function TibGains  = CombineTibGains(e0,G,loff,GSol,COMd)
% input arguments:

TibGains = [e0; G; loff; GSol; COMd];

== matlab function WEankle_controllerMaarten_TimingPerturb_2018/Ankle Controller/COMverror and perturbation/TriggerPerturbation/MATLAB Function2 ==
  data: Trigger output; SingleR input; SingleL input; PhaseL input; PhaseR input; GRFzL input; TypePert input; Delivered input
function Trigger   = Trigger(SingleR, SingleL, PhaseL, PhaseR, GRFzL, TypePert, Delivered)
%#codegen
% TypePert is vector with perturbations type 1-(Double stance rigth front) or 2-(middle left swing)
persistent i % index to go through TypePert vector
persistent delivered
persistent flagfirst %flag to indicate first time
if isempty(i)
    i = 1;
    flagfirst = 1;
end
delivered = Delivered;
if delivered == 1 && ~flagfirst %Perturbation delivered. Go to next element of TypePert avoiding a false entrance the first time
    i = i+1;
    delivered = 0; % not sure if neccessary 
end

len = length(TypePert);
if i > len %reset the index when all perturbations from the vector are done
    i = 1;
end
Pert = TypePert(i);

%%
Trigger = 0;
%% Left swing
% Left swing phase (SingleR == 1) -- Torque to right foot
if SingleR == 1    
    if ((10 <= PhaseR) && (PhaseR < 20)) && (Pert == 2)
        % Start left swing %TypePert=1
        Trigger = 1; 
    elseif ((20 <= PhaseR) && (PhaseR < 30)) && (Pert == 3)
        % mistance right leg
        Trigger = 1; 
    else
        Trigger = 0;
    end
end

%% Double stance (SingleR == 0 && SingleL == 0) -- Torques to both feet
if ((SingleR == 0) && (SingleL == 0))
   % Right in front - beginning of double stance %TypePert=1
   if ((0 <= PhaseR) && (PhaseR < 7) && (49 <= PhaseL) && (PhaseL < 60)) && (Pert == 1)
       Trigger = 1;
   else
       Trigger = 0;
   end
end
flagfirst = 0;

== matlab function WEankle_controllerMaarten_TimingPerturb_2018/Ankle Controller/MATLAB Function7 ==
  data: e0 input; G input; SolGains output; COMd input
function SolGains  = CombineSoleusGains(e0,G,COMd)
% input arguments:

SolGains = [e0; G; COMd];

== matlab function WEankle_controllerMaarten_TimingPerturb_2018/Ankle Controller/MATLAB Function8 ==
  data: e0 input; G input; loff input; GSol input; TibGains output; COMd input
function TibGains  = CombineTibGains(e0,G,loff,GSol,COMd)
% input arguments:

TibGains = [e0; G; loff; GSol; COMd];

== matlab function WEankle_controllerMaarten_TimingPerturb_2018/Ankle Controller/AnkleControllerGeyer1/ActivationDynamics1 ==
  data: e input; dadt output; a input
function dadt = ActDyn(e,a)

% See publication (DeGroote2016), equations 1-2, for more details
% (note tanh implementation mainly needed for gradient based optimization.
% Not needed in the actual controller. (I decided to keep it so that the
% dynamics of the parameter estimation and the controller are exactly the
% same

% tact = 0.02;
% tdeact = 0.04;

% contraction dynamics with smooth transition
% b = 0.001;
% d1 = 1./(tact.*(0.5+1.5*a));
% d2 = (0.5+1.5*a)./tdeact;
% f = 0.5*tanh(b*(e-a));
% dadt = (d1.*(f+0.5) + d2.*(-f+0.5)).*(e-a);

% try explicit version of contraction dynamics ( error in twincat with
% smooth version
% dadt = zeros(4,1);
% for i=1:length(a)
%     if a(i) < e(i)
%         tau_sel = tact;
%     else
%         tau_sel = tdeact;
%     end
%     dadt(i) = (e(i)-a(i))./ tau_sel;    
% end

% dadt = zeros(4,1);
% for i=1:length(a)   
%     dadt(i) = (e(i)-a(i))./ 0.03;    
% end

dadt = (e-a)./0.03;

== matlab function WEankle_controllerMaarten_TimingPerturb_2018/Ankle Controller/AnkleControllerGeyer1/ContractionDynamics1 ==
  data: a input; dlMdt output; lMtilde input; lMT input; F output; Fce_tilde output
function [dlMdt, F , Fce_tilde] = ContractionDynamics_Simulink(a,lMtilde,lMT)
% ContractionDynamics_Simulink Simulates contraction dynamics

% Muscle contraction dynamics left leg
[dlMdt_Left, F_Left , Fce_tilde_Left] = MuscleContractionDynamics(a(1:2),lMtilde(1:2),lMT(1:2));
 
% Muscle contraction dynamics right leg
[dlMdt_Right, F_Right , Fce_tilde_Right] = MuscleContractionDynamics(a(3:4),lMtilde(3:4),lMT(3:4));

% combine vectors
dlMdt = [dlMdt_Left; dlMdt_Right];
F = [F_Left; F_Right];
Fce_tilde = [Fce_tilde_Left; Fce_tilde_Right];
